simulink model "serialtest"  (R2014b)
settings: Solver=ode3  SolverMode=SingleTasking  StartTime=0.0  StopTime=inf  RelTol=1e-3
libraries: arduinolib x2
settings Model: SimulationMode=external  ExtModeTrigDuration=2  Creator=Edoardo  LastModifiedBy=Edoardo
settings OptimizationCC: OptimizeModelRefInitCode=on  LifeSpan=1
settings DebuggingCC: SolverPrmCheckMsg=none
settings HardwareCC: ProdBitPerInt=16  ProdBitPerPointer=8  ProdIntDivRoundTo=Zero  ProdEndianess=LittleEndian  ProdWordSize=8  ProdHWDeviceType=Atmel->AVR
settings RTWCC: SystemTargetFile=realtime.tlc  GenerateMakefile=off  TemplateMakefile=realtime.tmf  Description=Run on Target Hardware  RTWVerbose=off  ProcessScript=realtime_make_rtw_hook  IncludeHyperlinkInReport=on
settings STFCustomTargetCC: TargetLibSuffix=.a  GenerateSampleERTMain=on  ERTCustomFileBanners=on  SupportNonInlinedSFcns=off  SupportVariableSizeSignals=on  MATLABClassNameForMDSCustomization=Simulink.SoftwareTarget.ERTCustomization  GRTInterface=off  SystemTargetFile=realtime.tlc
settings ERTTargetCC: GenerateSampleERTMain=on  ParMdlRefBuildCompliant=off  CompOptLevelCompliant=off  ConcurrentExecutionCompliant=off  CombineOutputUpdateFcns=off  ERTFirstTimeCompliant=off  SupportContinuousTime=on  SupportVariableSizeSignals=on  ModelStepFunctionPrototypeControlCompliant=off  CPPClassGenCompliant=off  ExtMode=on  ExtModeTransport=3  ExtModeMexFile=ext_serial_win32_comm  ExtModeMexArgs=0 5 115200 30  InlinedParameterPlacement=NonHierarchical  ERTSrcFileBannerTemplate=realtime_code_template.cgt  ERTHdrFileBannerTemplate=realtime_code_template.cgt  ERTDataSrcFileTemplate=realtime_code_template.cgt  ERTDataHdrFileTemplate=realtime_code_template.cgt  ERTCustomFileTemplate=realtime_file_process.tlc

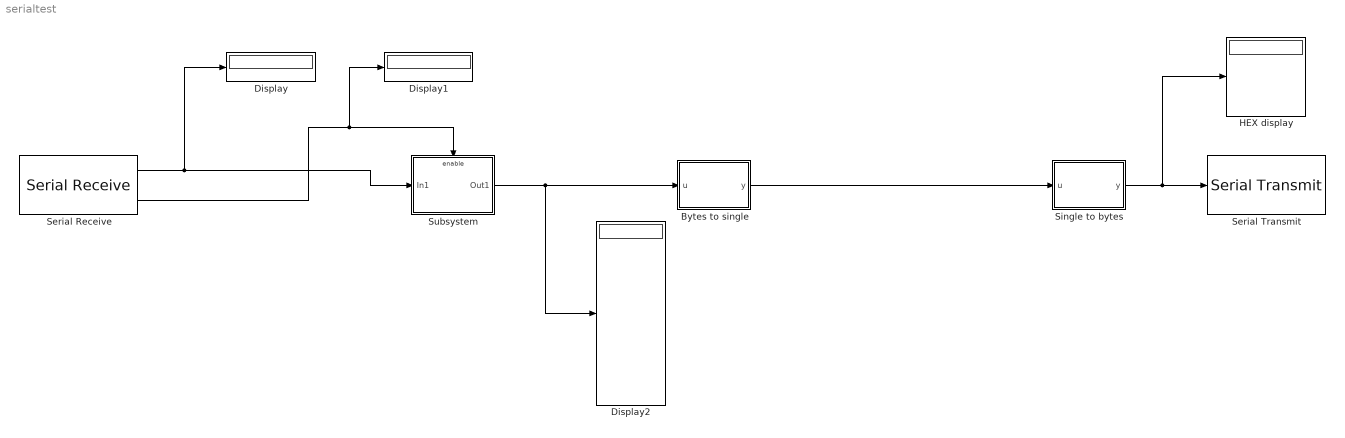
== system serialtest ==
  Bytes to single : MATLAB Function  TreatAsAtomicUnit=on
  Display : Display
  Display1 : Display
  Display2 : Display
      settings: Format=hex (Stored Integer)
  HEX display : Display
      settings: Format=hex (Stored Integer)
  Serial Receive : arduinolib/Serial Receive  portNumber=1  showOutStatus=on  sampleTime=0.1  blockPlatform=arduino
  Serial Transmit : arduinolib/Serial Transmit  portNumber=1  blockPlatform=arduino
  Single to bytes : MATLAB Function  TreatAsAtomicUnit=on
  Subsystem : Subsystem
  wires:
  Single to bytes/1(y) -> HEX display/1, Serial Transmit/1
  Bytes to single/1(y) -> Single to bytes/1(u)
  Serial Receive/1 -> Subsystem/1(In1), Display/1
  Serial Receive/2 -> Display1/1, Subsystem/Enable
  Subsystem/1(Out1) -> Display2/1, Bytes to single/1(u)

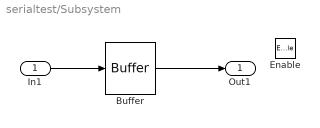
== system serialtest/Subsystem ==
  In1 : Inport
  Enable : EnablePort
  Buffer : Buffer  N=4  TreatMby1Signals=One channel
  Out1 : Outport
  wires:
  In1/1 -> Buffer/1
  Buffer/1 -> Out1/1

== matlab function serialtest/Bytes to single ==
  data: u input; y output size=1
function y = fcn(u)
%#codegen

s = typecast(u,'single');

y = s;

== matlab function serialtest/Single to bytes ==
  data: u input; y output size=4
function y = fcn(u)
%#codegen

b = typecast(single(u'),'uint8');

y = b';
